simulink subsystem "controls"  (R2022b)
settings: Solver=VariableStepAuto  StartTime=0.0  StopTime=10.0  RelTol=1e-3
settings Model: Creator=serga  LastModifiedBy=serga

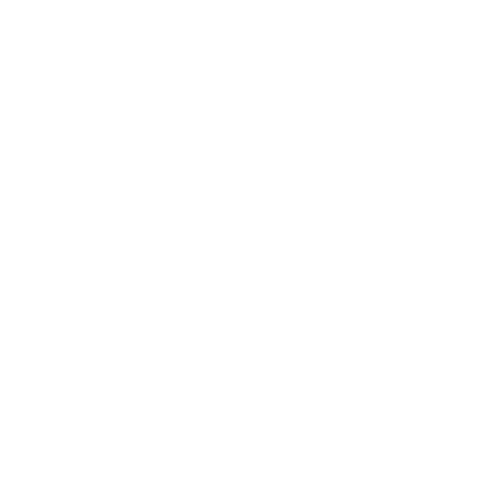
[thumbnail: Simulink's stored preview of the top-level diagram]
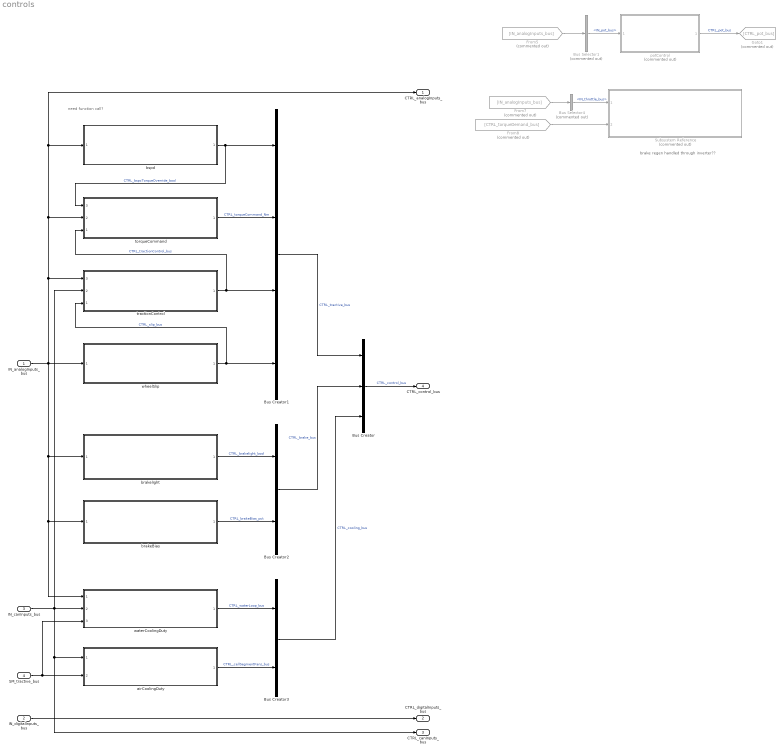
== system controls ==
  note: need function call?
  note: brake regen handled through inverter??
  IN_analogInputs_bus : Inport
  IN_digitalInputs_bus : Inport  Port=2
  IN_canInputs_bus : Inport  Port=3
  SM_tractive_bus : Inport  Port=4
  Bus Creator : BusCreator  Inputs=3
  Bus Creator1 : BusCreator  Inputs=4
  Bus Creator2 : BusCreator  Inputs=2
  Bus Creator3 : BusCreator  Inputs=2
  Bus Selector1 : BusSelector  Commented=on  OutputSignals=IN_pot_bus
  Bus Selector4 : BusSelector  Commented=on  OutputSignals=IN_throttle_bus
  From5 : From  Commented=on  GotoTag=IN_analogInputs_bus
  From7 : From  Commented=on  GotoTag=IN_analogInputs_bus
  From8 : From  Commented=on  GotoTag=CTRL_torqueDemand_bus
  Goto1 : Goto  Commented=on  GotoTag=CTRL_pot_bus
  Subsystem Reference : Subsystem  Commented=on  ReferencedSubsystem=brakeRegen
  airCoolingDuty : Subsystem  ReferencedSubsystem=airCoolingDuty
  brakeBias : Subsystem  ReferencedSubsystem=brakeBias
  brakelight : Subsystem  ReferencedSubsystem=brakelight
  bspd : Subsystem  ReferencedSubsystem=bspd
  potControl : Subsystem  Commented=on  ReferencedSubsystem=potControl
  torqueCommand : Subsystem  ReferencedSubsystem=torqueCommand
      settings: PortSchema="{\"entries\":[{\"content\":{\"sides\":[{\"content\":{\"connectorIds\":[\"In3\",\"In2\",\"In1\"]},\"type\":\"ConnectorPlacement.EquallySpacedRectSide\",\"uuid\":\"2c6e868d-198e-4fff-81f0-48170c11da3b\"},{\"content\":{\"connectorIds\":[\"Out1\"],\"side\":\"RIGHT\"},\"type\":\"ConnectorPlacement.EquallySpacedRectSide\",\"uuid\":\"7630e5d6-61c1-4c32-a26f-4ac5c7bab2a5\"},{\"content\":{\"connectorIds\":[],\"side\":\"TOP\"},\"type\":\"ConnectorPlacement.EquallySpacedRectSide\",\"uuid\":\"828693e2-a4de-4ae7-9f33-d4458fe7f3ed\"}]},\"type\":\"ConnectorPlacement.EquallySpacedConnector\",\"uuid\":\"e1e33393-9e12-493b-be33-d85b4e828102\"}],\"packageUris\":[\"http://schema.mathworks.com/mf0/Connector/R2020b\"],\"version\":\"1.0\"}"
  tractionControl : Subsystem  ReferencedSubsystem=tractionControl
      settings: PortSchema="{\"entries\":[{\"content\":{\"sides\":[{\"content\":{\"connectorIds\":[\"In3\",\"In2\",\"In1\"]},\"type\":\"ConnectorPlacement.EquallySpacedRectSide\",\"uuid\":\"2c6e868d-198e-4fff-81f0-48170c11da3b\"},{\"content\":{\"connectorIds\":[\"Out1\"],\"side\":\"RIGHT\"},\"type\":\"ConnectorPlacement.EquallySpacedRectSide\",\"uuid\":\"7630e5d6-61c1-4c32-a26f-4ac5c7bab2a5\"},{\"content\":{\"connectorIds\":[],\"side\":\"TOP\"},\"type\":\"ConnectorPlacement.EquallySpacedRectSide\",\"uuid\":\"828693e2-a4de-4ae7-9f33-d4458fe7f3ed\"}]},\"type\":\"ConnectorPlacement.EquallySpacedConnector\",\"uuid\":\"e1e33393-9e12-493b-be33-d85b4e828102\"}],\"packageUris\":[\"http://schema.mathworks.com/mf0/Connector/R2020b\"],\"version\":\"1.0\"}"
  waterCoolingDuty : Subsystem  ReferencedSubsystem=waterCoolingDuty
  wheelSlip : Subsystem  ReferencedSubsystem=wheelSlip
  CTRL_analogInputs_bus : Outport
  CTRL_digitalInputs_bus : Outport  Port=2
  CTRL_canInputs_bus : Outport  Port=3
  CTRL_control_bus : Outport  Port=4
  wires:
  From8/1 -> Subsystem Reference/2
  Bus Selector4/1 -> Subsystem Reference/1  "<IN_throttle_bus>"
  From7/1 -> Bus Selector4/1
  tractionControl/1 -> Bus Creator1/3, torqueCommand/1  "CTRL_tractionControl_bus"
  From5/1 -> Bus Selector1/1
  potControl/1 -> Goto1/1  "CTRL_pot_bus"
  Bus Selector1/1 -> potControl/1  "<IN_pot_bus>"
  wheelSlip/1 -> Bus Creator1/4, tractionControl/1  "CTRL_slip_bus"
  Bus Creator/1 -> CTRL_control_bus/1  "CTRL_control_bus"
  brakelight/1 -> Bus Creator2/1  "CTRL_brakelight_bool"
  brakeBias/1 -> Bus Creator2/2  "CTRL_brakeBias_pct"
  Bus Creator2/1 -> Bus Creator/2  "CTRL_brake_bus"
  Bus Creator1/1 -> Bus Creator/1  "CTRL_tractive_bus"
  torqueCommand/1 -> Bus Creator1/2  "CTRL_torqueCommand_Nm"
  IN_canInputs_bus/1 -> waterCoolingDuty/2, tractionControl/2, airCoolingDuty/1, CTRL_canInputs_bus/1
  IN_analogInputs_bus/1 -> brakeBias/1, waterCoolingDuty/1, brakelight/1, wheelSlip/1, torqueCommand/2, bspd/1, CTRL_analogInputs_bus/1, tractionControl/3
  bspd/1 -> Bus Creator1/1, torqueCommand/3  "CTRL_bspcTorqueOverride_bool"
  IN_digitalInputs_bus/1 -> CTRL_digitalInputs_bus/1
  SM_tractive_bus/1 -> airCoolingDuty/2, waterCoolingDuty/3
  waterCoolingDuty/1 -> Bus Creator3/1  "CTRL_waterLoop_bus"
  Bus Creator3/1 -> Bus Creator/3  "CTRL_cooling_bus"
  airCoolingDuty/1 -> Bus Creator3/2  "CTRL_cellSegmentFans_bus"
